simulink model "Schema_de_simulation_42"  (R2013a)
settings: Solver=ode45  StartTime=0.0  StopTime=12  RelTol=1e-3
values from neighbouring files (symbols this model uses):
  A = [-R/L 0 -Kc/L ... (first row only)    [lab03.m]
  B = [1/L ; 0 ; 0]    [lab03.m]
  B1 = 0.125    [lab03.m]
  Bm = 0.02    [lab03.m]
  C = [0 1 0]    [lab03.m]
  D = [0]    [lab03.m]
  g = 9.81    [lab03.m]
  J1 = 0.06    [lab03.m]
  Jm = 0.05    [lab03.m]
  Kc = 0.48    [lab03.m]
  Km = 0.5    [lab03.m]
  L = 0.00025    [lab03.m]
  l1 = 0.3    [lab03.m]
  M1 = 2    [lab03.m]
  perturbation_theta = 0    [lab03.m]
  perturbation_u = 0.05    [lab03.m]
  R = 0.5    [lab03.m]
settings Model: Creator=ToniO  LastModifiedBy=ToniO

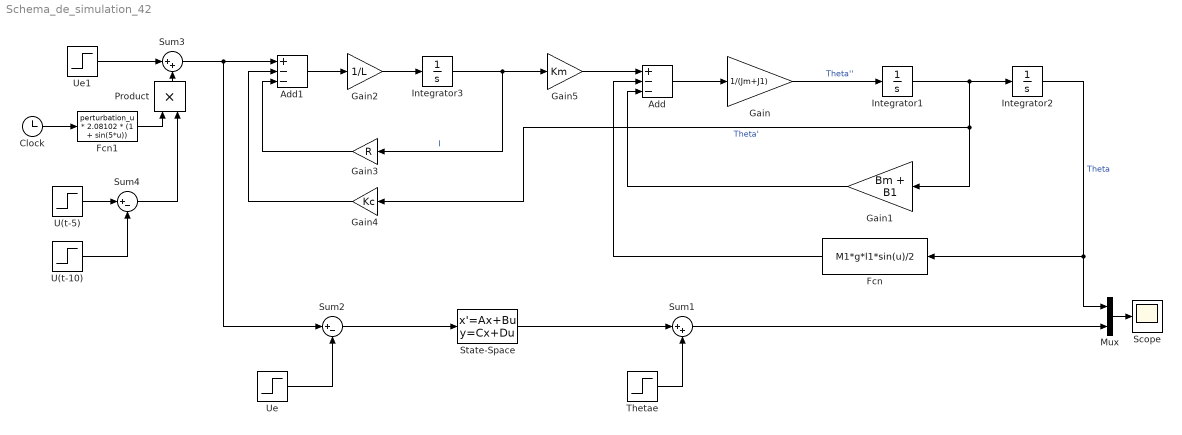
== system Schema_de_simulation_42 ==
  Add : Sum  Inputs=+--
  Add1 : Sum  Inputs=+--
  Clock : Clock
  Fcn : Fcn  Expr=M1*g*l1*sin(u)/2
  Fcn1 : Fcn  Expr=perturbation_u * 2.08102 * (1 + sin(5*u))
  Gain : Gain  Gain=1/(Jm+J1)
  Gain1 : Gain  Gain=Bm + B1
  Gain2 : Gain  Gain=1/L
  Gain3 : Gain  Gain=R
  Gain4 : Gain  Gain=Kc
  Gain5 : Gain  Gain=Km
  Integrator1 : Integrator
  Integrator2 : Integrator  InitialCondition=pi/4 + perturbation_theta*pi/180
  Integrator3 : Integrator  InitialCondition=4.16203
  Mux : Mux  Inputs=2
  Product : Product
  Scope : Scope
  State-Space : StateSpace  A=A  B=B  C=C  D=D  X0=perturbation_theta * pi / 180
  Sum1 : Sum  Inputs=|++
  Sum2 : Sum  Inputs=|+-
  Sum3 : Sum  Inputs=|++
  Sum4 : Sum  Inputs=|+-
  Thetae : Step  Time=0  After=pi/4  SampleTime=0
  U(t-10) : Step  Time=10  SampleTime=0
  U(t-5) : Step  Time=5  SampleTime=0
  Ue : Step  Time=0  Before=2.08102  After=2.08102  SampleTime=0
  Ue1 : Step  Time=0  Before=2.08102  After=2.08102  SampleTime=0
  wires:
  Add/1 -> Gain/1
  Integrator1/1 -> Gain4/1, Gain1/1, Integrator2/1  "Theta'"
  Integrator2/1 -> Mux/1, Fcn/1  "Theta"
  Gain/1 -> Integrator1/1  "Theta''"
  Gain1/1 -> Add/3
  Fcn/1 -> Add/2
  Add1/1 -> Gain2/1
  Gain2/1 -> Integrator3/1
  Integrator3/1 -> Gain5/1, Gain3/1  "I"
  Gain3/1 -> Add1/3
  Gain4/1 -> Add1/2
  Gain5/1 -> Add/1
  State-Space/1 -> Sum1/1
  Mux/1 -> Scope/1
  Sum2/1 -> State-Space/1
  Sum1/1 -> Mux/2
  Thetae/1 -> Sum1/2
  Ue/1 -> Sum2/2
  Clock/1 -> Fcn1/1
  Ue1/1 -> Sum3/1
  Sum3/1 -> Sum2/1, Add1/1
  Product/1 -> Sum3/2
  Fcn1/1 -> Product/1
  U(t-5)/1 -> Sum4/1
  U(t-10)/1 -> Sum4/2
  Sum4/1 -> Product/2
